simulink model "Model_til_jacob"  (R2015b)
settings: Solver=VariableStepAuto  StartTime=0.0  StopTime=10  RelTol=1e-3
values from neighbouring files (symbols this model uses):
  J_pro = (m*r^2+J_G2)*(G1/G2)^2 + J_G1    (= 0.281547798877)    [Control_Parameters.m]    (also in M_fil_til_jacob.m; PMSM_State_Space_Parameters.m)
  Kt = .07329    (= 0.07329)    [Control_Parameters.m]    (also in M_fil_til_jacob.m; PMSM_State_Space_Parameters.m)
  Kv = 0.001    [Control_Parameters.m]    (also in M_fil_til_jacob.m)
  L = 4e-5    (= 4e-05)    [Control_Parameters.m]    (also in M_fil_til_jacob.m; PMSM_State_Space_Parameters.m)
  R = .013/2    (= 0.0065)    [Control_Parameters.m]    (also in M_fil_til_jacob.m; PMSM_State_Space_Parameters.m)
settings Model: Creator=Morten  LastModifiedBy=Morten

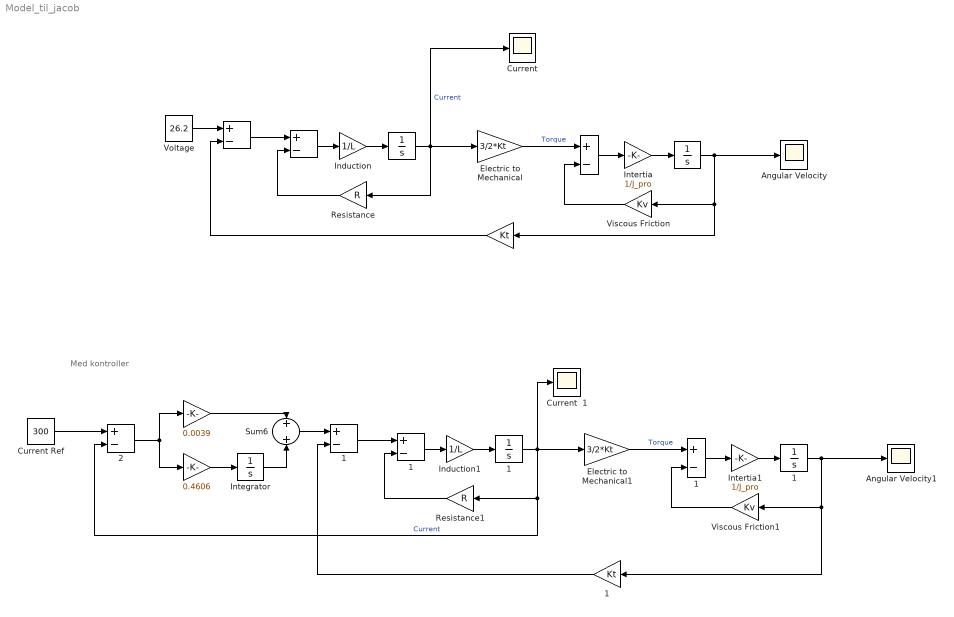
== system Model_til_jacob ==
  note: Med kontroller
  "  " : Sum  Inputs=+-
  "   " : Sum  Inputs=+-
  "    " : Sum  Inputs=+-
  " " : Gain  Gain=0.4606
  " " : Gain  Gain=0.0039
  "                          " : Integrator
  "                            " : Gain  Gain=Kt
  "                                     " : Integrator
  "                                     1" : Integrator
  "                            1" : Gain  Gain=Kt
  "                          1" : Integrator
  "    1" : Sum  Inputs=+-
  "   1" : Sum  Inputs=+-
  "  1" : Sum  Inputs=+-
  "  2" : Sum  Inputs=+-
  Angular Velocity : Scope
  Angular Velocity1 : Scope
  "Current  " : Scope
  Current  1 : Scope
  Current Ref : Constant  Value=300
  Electric to Mechanical : Gain  Gain=3/2*Kt
  Electric to Mechanical1 : Gain  Gain=3/2*Kt
  Induction : Gain  Gain=1/L
  Induction1 : Gain  Gain=1/L
  Integrator : Integrator
  Intertia : Gain  Gain=1/J_pro
  Intertia1 : Gain  Gain=1/J_pro
  Resistance : Gain  Gain=R
  Resistance1 : Gain  Gain=R
  Sum6 : Sum
  Viscous Friction : Gain  Gain=Kv
  Viscous Friction1 : Gain  Gain=Kv
  Voltage : Constant  Value=26.2
  wires:
  "  "/1 -> "   "/1
  "   "/1 -> Induction/1
  Induction/1 -> "                          "/1
  Resistance/1 -> "   "/2
  "                          "/1 -> Resistance/1, Electric to Mechanical/1, "Current  "/1  "Current"
  "    "/1 -> Intertia/1
  Intertia/1 -> "                                     "/1
  "                            "/1 -> "  "/2
  Voltage/1 -> "  "/1
  "                                     "/1 -> Angular Velocity/1, "                            "/1, Viscous Friction/1
  Electric to Mechanical/1 -> "    "/1  "Torque"
  Viscous Friction/1 -> "    "/2
  "  1"/1 -> "   1"/1
  "   1"/1 -> Induction1/1
  Induction1/1 -> "                          1"/1
  Resistance1/1 -> "   1"/2
  "                          1"/1 -> "  2"/2, Resistance1/1, Electric to Mechanical1/1, Current  1/1  "Current"
  "    1"/1 -> Intertia1/1
  Intertia1/1 -> "                                     1"/1
  "                            1"/1 -> "  1"/2
  "                                     1"/1 -> Angular Velocity1/1, "                            1"/1, Viscous Friction1/1
  Electric to Mechanical1/1 -> "    1"/1  "Torque"
  Viscous Friction1/1 -> "    1"/2
  Current Ref/1 -> "  2"/1
  "  2"/1 -> " "/1, " "/1
  " "/1 -> Sum6/1
  " "/1 -> Integrator/1
  Integrator/1 -> Sum6/2
  Sum6/1 -> "  1"/1
